simulink library "Project4_lib_2015b"  (R2015b)
settings: Solver=VariableStepAuto  SolverMode=SingleTasking  StartTime=0.0  StopTime=10.0  RelTol=1e-3
values from neighbouring files (symbols this model uses):
  C1 = 3.5e4    (= 35000)    [init.m]
  Q = Capacity*3600    (= 111600)    [init.m]
  R0 = 0.009    [init.m]
  R1 = 0.0015    [init.m]
libraries: simulink x2, simulink_extras x1
settings Model: Creator=wasynczu  LastModifiedBy=wasynczu
settings DataIOCC: LimitDataPoints=off
settings DebuggingCC: AllowSymbolicDim=on  SFUnexpectedBacktrackingDiag=error  SFNoUnconditionalDefaultTransitionDiag=error
settings ModelReferenceCC: PropagateSignalLabelsOutOfModel=on
settings SFSimCC: SimUseLocalCustomCode=on
settings RTWCC: RTWUseLocalCustomCode=on
settings GRTTargetCC: TargetLangStandard=C99 (ISO)
settings ConfigComp: CovMetricSettings=dwe  CovHtmlReporting=off  CovSaveCumulativeToWorkspaceVar=off  CovSaveSingleToWorkspaceVar=off  CovModelRefEnable=Off  CovExternalEMLEnable=on

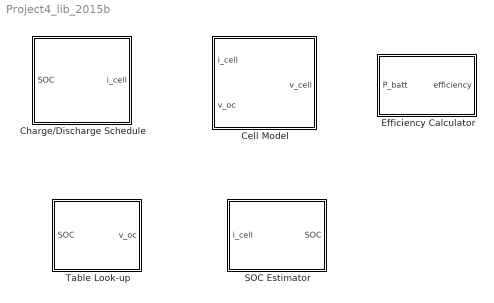
== system Project4_lib_2015b ==
  Cell Model : Subsystem  mask{R0=R0, R1=R1, C1=C1}
  Charge/Discharge Schedule : Subsystem  mask{c_rate_charge=0.2, c_rate_discharge=0.2, SOC_max=1, SOC_min=0.2}
  Efficiency Calculator : Subsystem
  SOC Estimator : Subsystem  mask{SOC_init=0.2}
  Table Look-up : Subsystem

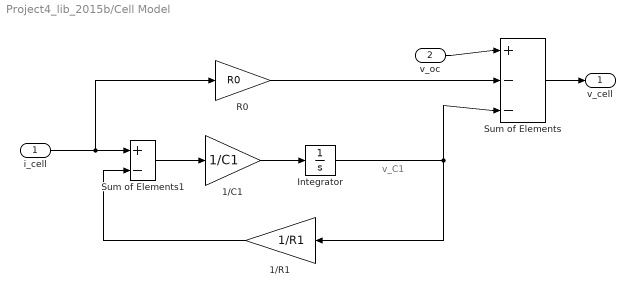
== system Project4_lib_2015b/Cell Model ==
  note: v_C1
  i_cell : Inport
  "v_oc " : Inport  Port=2
  1/C1 : Gain  Gain=1/C1
  1/R1 : Gain  Gain=1/R1
  Integrator : Integrator
  R0 : Gain  Gain=R0
  Sum of Elements : Sum  Inputs=+--
  Sum of Elements1 : Sum  Inputs=+-
  v_cell : Outport
  wires:
  i_cell/1 -> R0/1, Sum of Elements1/1
  "v_oc "/1 -> Sum of Elements/1
  R0/1 -> Sum of Elements/2
  Sum of Elements1/1 -> 1/C1/1
  1/C1/1 -> Integrator/1
  Sum of Elements/1 -> v_cell/1
  1/R1/1 -> Sum of Elements1/2
  Integrator/1 -> 1/R1/1, Sum of Elements/3

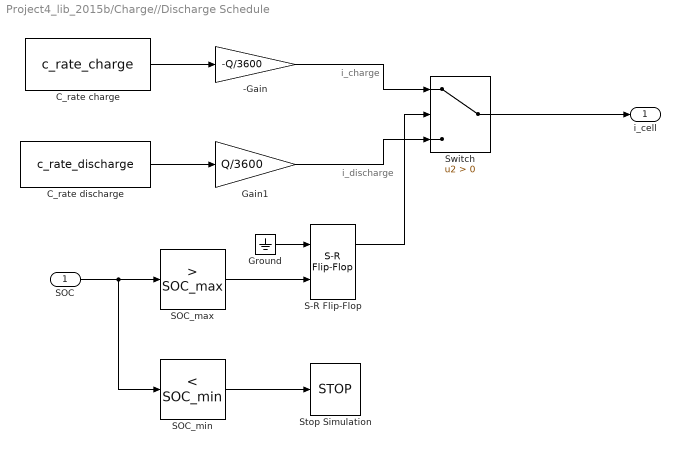
== system Project4_lib_2015b/Charge//Discharge Schedule ==
  note: i_discharge
  note: i_charge
  SOC : Inport
  -Gain : Gain  Gain=-Q/3600
  C_rate charge : Constant  Value=c_rate_charge
  C_rate discharge : Constant  Value=c_rate_discharge
  Gain1 : Gain  Gain=Q/3600
  Ground : Ground
  S-R Flip-Flop : simulink_extras/Flip Flops/S-R Flip-Flop  initial_condition=1
  "SOC_max " : simulink/Logic and Bit Operations/Compare To Constant  relop=>  const=SOC_max  OutDataTypeStr=boolean
  SOC_min : simulink/Logic and Bit Operations/Compare To Constant  relop=<  const=SOC_min  OutDataTypeStr=boolean
  Stop Simulation : Stop
  Switch : Switch  Criteria=u2 > Threshold
  "i_cell " : Outport
  wires:
  C_rate charge/1 -> -Gain/1
  C_rate discharge/1 -> Gain1/1
  -Gain/1 -> Switch/1
  Gain1/1 -> Switch/3
  S-R Flip-Flop/1 -> Switch/2
  "SOC_max "/1 -> S-R Flip-Flop/2
  SOC/1 -> SOC_min/1, "SOC_max "/1
  SOC_min/1 -> Stop Simulation/1
  Switch/1 -> "i_cell "/1
  Ground/1 -> S-R Flip-Flop/1

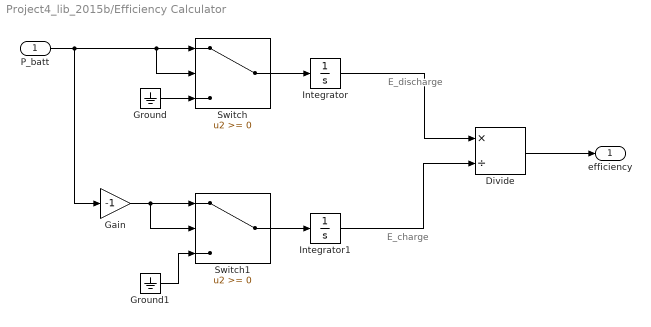
== system Project4_lib_2015b/Efficiency Calculator ==
  note: E_charge
  note: E_discharge
  P_batt : Inport
  Divide : Product  Inputs=*/
  Gain : Gain  Gain=-1
  Ground : Ground
  Ground1 : Ground
  Integrator : Integrator
  Integrator1 : Integrator
  Switch : Switch
  Switch1 : Switch
  efficiency : Outport
  wires:
  P_batt/1 -> Gain/1, Switch/2, Switch/1
  Ground/1 -> Switch/3
  Gain/1 -> Switch1/2, Switch1/1
  Ground1/1 -> Switch1/3
  Switch/1 -> Integrator/1
  Switch1/1 -> Integrator1/1
  Integrator/1 -> Divide/1
  Integrator1/1 -> Divide/2
  Divide/1 -> efficiency/1

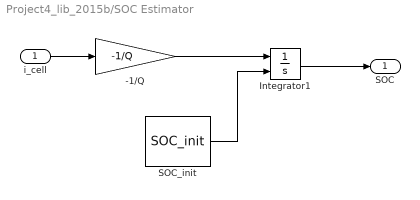
== system Project4_lib_2015b/SOC Estimator ==
  i_cell : Inport
  -1/Q : Gain  Gain=-1/Q
  Integrator1 : Integrator  InitialConditionSource=external
  SOC_init : Constant  Value=SOC_init
  SOC : Outport
  wires:
  i_cell/1 -> -1/Q/1
  -1/Q/1 -> Integrator1/1
  Integrator1/1 -> SOC/1
  SOC_init/1 -> Integrator1/2

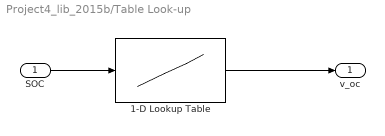
== system Project4_lib_2015b/Table Look-up ==
  SOC : Inport
  1-D Lookup Table : Lookup_n-D  NumberOfTableDimensions=1  BreakpointsForDimension1=[0 0.1 0.25 0.5 0.75 0.9 1]  Table="[ 3.51  3.57  3.63  3.71  3.93  4.08  4.19]"  RndMeth=Simplest  InputSameDT=on
  v_oc : Outport
  wires:
  SOC/1 -> 1-D Lookup Table/1
  1-D Lookup Table/1 -> v_oc/1
